simulink model "PROGRAMMING_EXERCISE_PART9_1"  (R2017b)
settings: Solver=VariableStepAuto  StartTime=0.0  StopTime=3  RelTol=1e-3
settings Model: Creator=chenjiasheng  LastModifiedBy=chenjiasheng

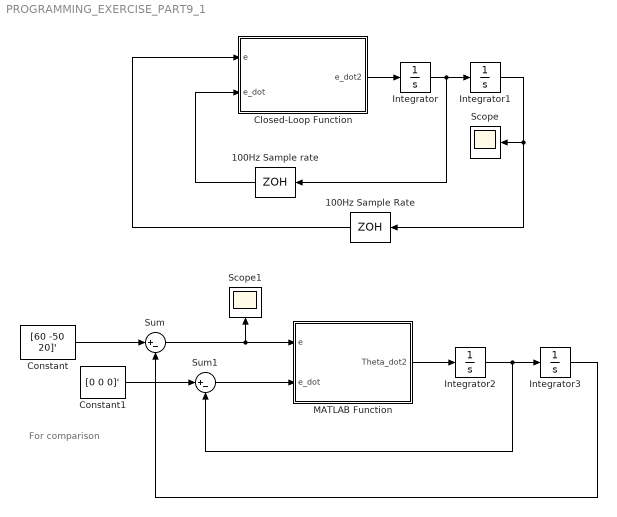
== system PROGRAMMING_EXERCISE_PART9_1 ==
  note: For comparison
  100Hz Sample Rate : ZeroOrderHold  SampleTime=0.01
  100Hz Sample rate : ZeroOrderHold  SampleTime=0.01
  Closed-Loop Function : MATLAB Function  TreatAsAtomicUnit=on
  Constant : Constant  Value=[60 -50 20]'
  Constant1 : Constant  Value=[0 0 0]'
  Integrator : Integrator  InitialCondition=[0 0 0]'
  Integrator1 : Integrator  InitialCondition=[0 60 0]'
  Integrator2 : Integrator  InitialCondition=[0 0 0]'
  Integrator3 : Integrator  InitialCondition=[60 -110 20]'
  MATLAB Function : MATLAB Function  TreatAsAtomicUnit=on
  Scope : Scope
  Scope1 : Scope
  Sum : Sum  Inputs=|+-
  Sum1 : Sum  Inputs=|+-
  wires:
  Closed-Loop Function/1(e_dot2) -> Integrator/1
  Integrator/1 -> 100Hz Sample rate/1, Integrator1/1
  Integrator1/1 -> Scope/1, 100Hz Sample Rate/1
  MATLAB Function/1(Theta_dot2) -> Integrator2/1
  Integrator2/1 -> Integrator3/1, Sum1/2
  Integrator3/1 -> Sum/2
  Constant/1 -> Sum/1
  Sum/1 -> Scope1/1, MATLAB Function/1(e)
  Sum1/1 -> MATLAB Function/2(e_dot)
  Constant1/1 -> Sum1/1
  100Hz Sample rate/1 -> Closed-Loop Function/2(e_dot)
  100Hz Sample Rate/1 -> Closed-Loop Function/1(e)

== matlab function PROGRAMMING_EXERCISE_PART9_1/MATLAB Function ==
  data: e input; Theta_dot2 output; e_dot input
function Theta_dot2 = fcn(e,e_dot)
Theta_dot2=[175 0   0;
            0   110 0;
            0   0   20]*e+[2*sqrt(175) 0           0;
                           0           2*sqrt(110) 0;
                           0           0           2*sqrt(20)]*e_dot
end

== matlab function PROGRAMMING_EXERCISE_PART9_1/Closed-Loop Function ==
  data: e input; e_dot2 output; e_dot input
function e_dot2 = fcn(e,e_dot)
e_dot2=-[175 0   0;
         0   110 0;
         0   0   20]*e-[2*sqrt(175) 0           0;
                        0           2*sqrt(110) 0;
                        0           0           2*sqrt(20)]*e_dot;
end
